simulink library "system_blocks"  (Simulink 8.4)
settings: Solver=ode45  SolverMode=SingleTasking  StartTime=0.0  StopTime=10.0  RelTol=1e-3
values from neighbouring files (symbols this model uses):
  A = 'STP1'    [digital_communications_gui.m]
  D = 'STP4'    [digital_communications_gui.m]
  T = 273+20    (= 293)    [exercise_00.m]
undefined symbols (not defined in the file or in its folder): T4
libraries: simulink x9, dspswit3 x5, dspsigops x2, dspobslib x2, dsparch4 x1, simulink_extras x1, dspmtrx3 x1
(part 1 of 2)
settings Model: Creator=Schoenen  LastModifiedBy=Schoenen

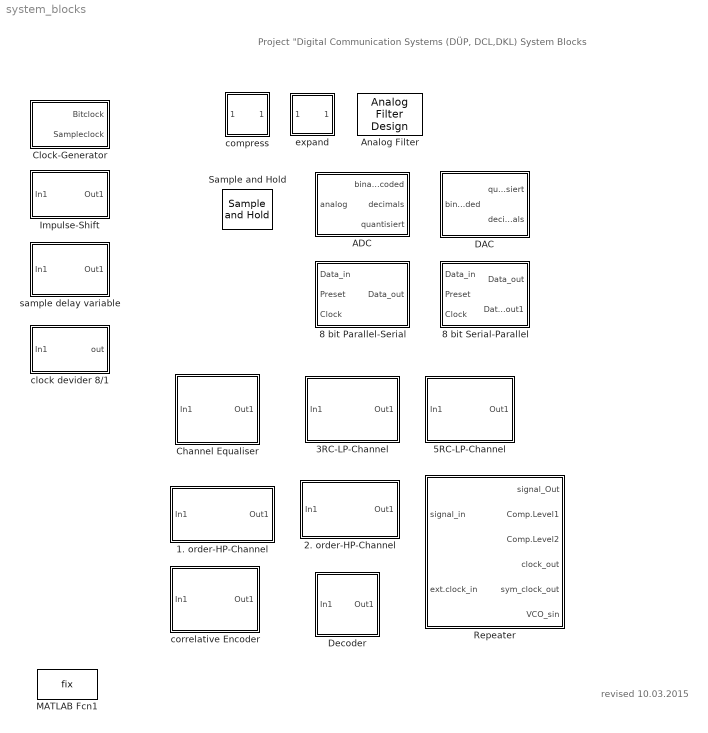
== system system_blocks ==
  note: revised 10.03.2015
  note: Project "Digital Communication Systems (DÜP, DCL,DKL)
      | System Blocks
  1. order-HP-Channel : Subsystem  mask{grenz=400}
      mask prompts: grenz "3 dB-Cutoff frequency (Hz):"
      mask help: Hochpass 1. Ordnung mit wählbarer Grenzfrequenz
      mask init:
      | if grenz==1 T=1/(2*pi*400); end;
      | if grenz==2 T=1/(2*pi*2e3); end;
      | if grenz==3 T=1/(2*pi*3e3); end;
      mask TypeOptions grenz: 400 | 2e3 | 3e3
  2. order-HP-Channel : Subsystem  mask{grenz=400}
      mask prompts: grenz "3 dB-Cutoff frequency (Hz):"
      mask help: Hochpass 2. Ordnung mit wählbarer Grenzfrequenz
      mask init:
      | if grenz==1 T=1/(2*pi*400)*1.554; end;
      | if grenz==2 T=1/(2*pi*2e3)*1.554; end;
      | if grenz==3 T=1/(2*pi*3e3)*1.554; end;
      mask TypeOptions grenz: 400 | 2e3 | 3e3
  "3RC-LP-Channel " : Subsystem  mask{noise=0.1, a=off, step=2/64e5}
      mask prompts: noise "Noise (rms):"; a "Noise on"; step "Simulation Step size:"
      mask help: Kanalmodell mit 3 RC-Gliedern und additivem Rauschen
      mask init:
      | T=10e3*159e-12;
  "5RC-LP-Channel " : Subsystem  mask{noise=0.1, a=off, step=2/64e5}
      mask prompts: noise "Noise (rms):"; a "Noise on"; step "Simulation Step size:"
      mask help: Kanalmodell mit 5 RC-Gliedern und additivem Rauschen
      mask init:
      | T=10e3*159e-12;
  8 bit Parallel-Serial : Subsystem
  8 bit Serial-Parallel : Subsystem
  ADC : Subsystem  mask(Analog-Digital-Converter (ADC)){umax=1, bits=1, bipolar=off}
      mask prompts: umax "Aussteuergrenze:"; bits "Bitanzahl (1...16):"; bipolar "Bipolares binäres Ausgangssignal (binary_coded)"
      mask help:
      | Der ADC wandelt ein bipolares Analogsignal mit den Austeuergrenzen +/- Umax in ein Digitalsignal entsprechender Bitzahl (PCM) um.
      |
      | Oberer Ausgang:      Bit-Parallel-Ausgang, Binäre Zahlenfolge, je Abtastwert ein Zeilenvektor in Binärdarstellung
      |
      | Mittlerer Ausgang:   dem Eingang entsprechender quantisierter positiver Dezimalwert im Bereich 0.... 2^bits -1
      |
      | Unterer Ausgang:    Quantisiertes, bipolares Signal, begrenzt auf +/- Umax, je Abtastwert ein als Skalar
      mask Help:
      | Author: Prof. Dr.-Ing. Peter Kröger
      | copyright 2002
      | <p>
      | Der ADC wandelt ein bipolares Analogsignal mit den Austeuergrenzen +/- Umax in ein Digitalsignal entsprechender Bitzahl (PCM-Signal) um.
      | <p>
      | Oberer Ausgang:     Binäre Zahlenfolge, je Abtastwert ein Zeilenvektor in
      |                                 Binärdarstellung
      | <p>
      | Mittlerer Ausgang:   dem Eingang entsprechender quantisierter positiver                                           Dezimalwert im Bereich 0.... 2^bits -1
      | <p>
      | Unterer Ausgang:    Quantisiertes, bipolares Signal, begrenzt auf +/- Umax,
      |                              je Abtastwert ein als Skalar
  Analog Filter : dsparch4/Analog Filter Design  method=Butterworth  filttype=Lowpass  N=1  Wlo=1  Whi=80  Rp=2  Rs=40
  Channel Equaliser : Subsystem
  Clock-Generator : Subsystem  mask{bt=1, sr=1}
      mask prompts: bt "Bitclock (Hz):"; sr "Sampleclock (Hz):"
      mask help: Clock-Generator
  DAC : Subsystem  mask(Digital-Analog-Converter (DAC)){umax=1, bits=1, bipolar=off}
      mask prompts: umax "maximum voltage limit"; bits "number of bits (1...16)"; bipolar "bipolar binary input sequence"
      mask help:
      | Der DAC wandelt ein binäres Digitalsignal (PCM) in ein bipolares, quantisiertes Analogsignal mit den Austeuergrenzen +/- Umax um.
      |
      | Eingang :              Bit-Paralleleingang, Binäre PCM-Zahlenfolge, je Abtastwert ein Zeilenvektor in Binärdarstellung
      |
      | Oberer  Ausgang:   Quantisiertes, bipolares Signal, begrenzt auf +/- Umax,  je Abtastwert ein als Skalar
      |
      | Unterer Ausgang:   dem Eingang entsprechender positiver  Dezimalwert im Bereich 0.... 2^bits -1
      mask Help:
      | Author: Prof. Dr.-Ing. Peter Kröger
      | copyright 2002
      | <p>
      | 
      | Der DAC wandelt ein binäres Digitalsignal (PCM) in ein bipolares, quantisiertes Analogsignal mit den Austeuergrenzen +/- Umax um.
      | <p>
      | Eingang :                Binäre PCM-Zahlenfolge, je Abtastwert ein Zeilenvektor in
      |                                Binärdarstellung
      | <p>
      | Oberer  Ausgang:   Quantisiertes, bipolares Signal, begrenzt auf +/- Umax,
      |                                je Abtastwert ein als Skalar
      | <p>
      | Unterer Ausgang:   dem Eingang entsprechender positiver  Dezimalwert
      |                                im Bereich 0.... 2^bits -1
  Decoder : Subsystem
  Impulse-Shift : Subsystem  mask{tau=1, width=1, step=2/64e5}
      mask prompts: tau "Phase-Shift [s]"; width "output impulse-width [s]"; step "Simulation Stepsize [s]"
      mask help:
      | Impulse Shift.
      |
      | The Block is triggered on positive edge at input and answers with an output impulse later correspopnding to the Parameter "Phase Shift".
      | The width of the output impuls can be varied.
      | If periodic triggering is applied to the block, the Phase Shift must be less than the trigger period.
  MATLAB Fcn1 : MATLABFcn  MATLABFcn=fix  OutputDimensions=1
  Repeater : Subsystem
  Sample and Hold : dspsigops/Sample and Hold  trig=Rising edge  initCond=0  latchinput=off
  clock devider 8/1 : Subsystem  mask{bt=1, sr=1}
      mask prompts: bt "Bitclock [Hz]"; sr "Sampleclock [Hz]"
      mask help: Clock-Generator
  compress : Subsystem  mask{ck=16}
      mask prompts: ck "comp. factor ck"
      mask help:
      | A-law-compression
      | ck=1	->	 A=1
      | ck=2	->	 A=5.36
      | ck=4	->	 A=14.77
      | ck=8	->	 A=36.85
      | ck=16	->	A=87.56  (ISDN)
      | ck=32	->	A=201.84
      mask init:
      | if ck==1, A=1;
      | 	elseif ck==2, A=5.36;
      | 	elseif ck==4, A=14.77;
      | 	elseif ck==8, A=36.85;
      | 	elseif ck==16, A=87.56;
      | 	else A=201.84;
      | 	end;
      | 	
      | x=-1:.01:1;
      | for i=1:201, 
      | 	if abs(x(i))<1/A, y(i)=ck*x(i); 
      | 	else y(i) = sign(x(i))*(1+log(A*abs(x(i))))/(1+log(A)); 
      | 	end; 
      | end;
      mask Display: plot(x,y)
  correlative Encoder : Subsystem
  expand : Subsystem  mask{ck=16}
      mask prompts: ck "comp. factor ck"
      mask help:
      | A-law-expansion
      | ck=1	->	 A=1
      | ck=2	->	 A=5.36
      | ck=4	->	 A=14.77
      | ck=8	->	 A=36.85
      | ck=16	->	A=87.56  (ISDN)
      | ck=32	->	A=201.84
      mask init:
      | if ck==1, A=1;
      | 	elseif ck==2, A=5.36;
      | 	elseif ck==4, A=14.77;
      | 	elseif ck==8, A=36.85;
      | 	elseif ck==16, A=87.56;
      | 	else A=201.84;
      | 	end;
      | 
      | x=-1:.01:1;
      | for i=1:201,
      | 	if abs(x(i))<ck/A, y(i) = x(i)/ck;
      | 	else y(i) = sign(x(i))*(exp((1+log(A))*abs(x(i)) - 1))/A;
      | 	end;
      | end;
      mask Display: plot(x,y)
  sample delay variable : Subsystem

== system system_blocks/1. order-HP-Channel ==
  In1 : Inport
  HP-1.Ordnung : TransferFcn  Numerator=[T 0]  Denominator=[T 1]
  Out1 : Outport
  wires:
  HP-1.Ordnung/1 -> Out1/1
  In1/1 -> HP-1.Ordnung/1

== system system_blocks/2. order-HP-Channel ==
  In1 : Inport
  HP-1.Ordnung : TransferFcn  Numerator=[T^2 0 0]  Denominator=[T^2 2*T 1]
  Out1 : Outport
  wires:
  HP-1.Ordnung/1 -> Out1/1
  In1/1 -> HP-1.Ordnung/1

== system system_blocks/3RC-LP-Channel  ==
  In1 : Inport
  3 RC-Glieder : TransferFcn  Denominator=[T^3 5*T^2 6*T 1]
  Band-Limited White Noise : Subsystem  mask(Continuous White Noise.){Cov=[noise^2*step], Ts=step, seed=[23341]}
      mask prompts: Cov "Noise Power:"; Ts "Sample Time:"
      mask help:
      | White noise for continuous (s-domain) systems.
      | Band-limited using zero-order-hold.
      mask init:
      | r = rand(1,12); r2 = [r(1),r;r,r(12)]; t =[1:13;1:13];
      mask Help: Implemented using white noise into Zero-Order Hold block. The seed and power can be vectors of the same length to produce a vector of white noise sources. For faster simulation, set sample time to the highest value possible but in accordance with the fastest dynamics of system.
      mask Display: plot(t(:),r2(:))
  Constant : Constant  Value=a
  Ground : Ground
  Sum2 : Sum  SaturateOnIntegerOverflow=on  InputSameDT=on  OutDataTypeStr=Inherit: Same as first input
  Switch : Switch  Threshold=0.5  SaturateOnIntegerOverflow=on
  Out1 : Outport
  wires:
  Ground/1 -> Switch/3
  Constant/1 -> Switch/2
  3 RC-Glieder/1 -> Sum2/1
  Band-Limited White Noise/1(Out_1) -> Switch/1
  In1/1 -> 3 RC-Glieder/1
  Switch/1 -> Sum2/2
  Sum2/1 -> Out1/1

== system system_blocks/5RC-LP-Channel  ==
  In1 : Inport
  5 RC-Glieder : TransferFcn  Denominator=[T^5 9*T^4 28*T^3 35*T^2 15*T 1]
  Band-Limited White Noise : Subsystem  mask(Continuous White Noise.){Cov=[noise^2*step], Ts=step, seed=[23341]}
      mask prompts: Cov "Noise Power:"; Ts "Sample Time:"
      mask help:
      | White noise for continuous (s-domain) systems.
      | Band-limited using zero-order-hold.
      mask init:
      | r = rand(1,12); r2 = [r(1),r;r,r(12)]; t =[1:13;1:13];
      mask Help: Implemented using white noise into Zero-Order Hold block. The seed and power can be vectors of the same length to produce a vector of white noise sources. For faster simulation, set sample time to the highest value possible but in accordance with the fastest dynamics of system.
      mask Display: plot(t(:),r2(:))
  Constant : Constant  Value=a
  Ground : Ground
  Sum2 : Sum  SaturateOnIntegerOverflow=on  InputSameDT=on  OutDataTypeStr=Inherit: Same as first input
  Switch : Switch  Threshold=0.5  SaturateOnIntegerOverflow=on
  Out1 : Outport
  wires:
  Ground/1 -> Switch/3
  Constant/1 -> Switch/2
  5 RC-Glieder/1 -> Sum2/1
  Band-Limited White Noise/1(Out_1) -> Switch/1
  In1/1 -> 5 RC-Glieder/1
  Switch/1 -> Sum2/2
  Sum2/1 -> Out1/1

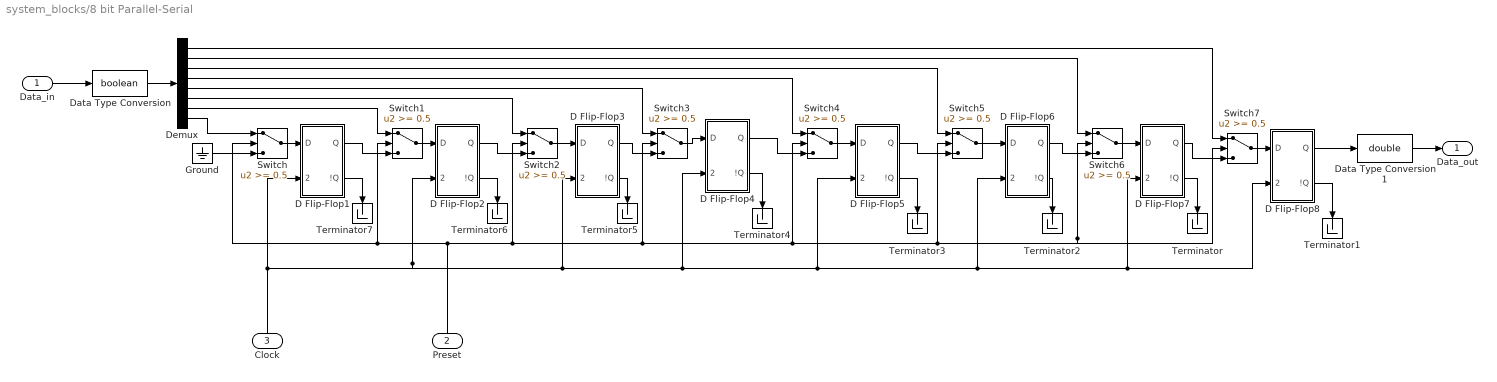
== system system_blocks/8 bit Parallel-Serial ==
  Data_in : Inport
  Preset : Inport  Port=2
  Clock : Inport  Port=3
  D Flip-Flop1 : Subsystem  AncestorBlock=simulink_extras/Flip Flops/D Flip-Flop  mask(DFlipFlop){}
      mask help: D Flip-Flop Block
      mask Help:
      | The D flip-flop block has the following characteristic table:
      | <pre>
      |   Q(t)  D(t)     Q(tnext)
      |   ------------------------
      |    0      0       0
      |    0      1       1
      |    1      0       0
      |    1      1       1
      | </pre>
      | Q(tnext) refers to the output on a clock pulse (CLK) rising edge and when the
      | chip is enabled (!CLR ~= 0).
      | <br><br>
      | The D flip-flop transfers "data" into a memory element (flip-flop) on each clock
      | pulse (CLK). The chip enable input signal, !CLR, is sometimes given the
      | designation G (for gate) to indicate that this input enables the gated latch
      | allowing data entry into the flip-flop.
  D Flip-Flop2 : Subsystem  AncestorBlock=simulink_extras/Flip Flops/D Flip-Flop  mask(DFlipFlop){}
      mask help: D Flip-Flop Block
      mask Help:
      | The D flip-flop block has the following characteristic table:
      | <pre>
      |   Q(t)  D(t)     Q(tnext)
      |   ------------------------
      |    0      0       0
      |    0      1       1
      |    1      0       0
      |    1      1       1
      | </pre>
      | Q(tnext) refers to the output on a clock pulse (CLK) rising edge and when the
      | chip is enabled (!CLR ~= 0).
      | <br><br>
      | The D flip-flop transfers "data" into a memory element (flip-flop) on each clock
      | pulse (CLK). The chip enable input signal, !CLR, is sometimes given the
      | designation G (for gate) to indicate that this input enables the gated latch
      | allowing data entry into the flip-flop.
  D Flip-Flop3 : Subsystem  AncestorBlock=simulink_extras/Flip Flops/D Flip-Flop  mask(DFlipFlop){}
      mask help: D Flip-Flop Block
      mask Help:
      | The D flip-flop block has the following characteristic table:
      | <pre>
      |   Q(t)  D(t)     Q(tnext)
      |   ------------------------
      |    0      0       0
      |    0      1       1
      |    1      0       0
      |    1      1       1
      | </pre>
      | Q(tnext) refers to the output on a clock pulse (CLK) rising edge and when the
      | chip is enabled (!CLR ~= 0).
      | <br><br>
      | The D flip-flop transfers "data" into a memory element (flip-flop) on each clock
      | pulse (CLK). The chip enable input signal, !CLR, is sometimes given the
      | designation G (for gate) to indicate that this input enables the gated latch
      | allowing data entry into the flip-flop.
  D Flip-Flop4 : Subsystem  AncestorBlock=simulink_extras/Flip Flops/D Flip-Flop  mask(DFlipFlop){}
      mask help: D Flip-Flop Block
      mask Help:
      | The D flip-flop block has the following characteristic table:
      | <pre>
      |   Q(t)  D(t)     Q(tnext)
      |   ------------------------
      |    0      0       0
      |    0      1       1
      |    1      0       0
      |    1      1       1
      | </pre>
      | Q(tnext) refers to the output on a clock pulse (CLK) rising edge and when the
      | chip is enabled (!CLR ~= 0).
      | <br><br>
      | The D flip-flop transfers "data" into a memory element (flip-flop) on each clock
      | pulse (CLK). The chip enable input signal, !CLR, is sometimes given the
      | designation G (for gate) to indicate that this input enables the gated latch
      | allowing data entry into the flip-flop.
  D Flip-Flop5 : Subsystem  AncestorBlock=simulink_extras/Flip Flops/D Flip-Flop  mask(DFlipFlop){}
      mask help: D Flip-Flop Block
      mask Help:
      | The D flip-flop block has the following characteristic table:
      | <pre>
      |   Q(t)  D(t)     Q(tnext)
      |   ------------------------
      |    0      0       0
      |    0      1       1
      |    1      0       0
      |    1      1       1
      | </pre>
      | Q(tnext) refers to the output on a clock pulse (CLK) rising edge and when the
      | chip is enabled (!CLR ~= 0).
      | <br><br>
      | The D flip-flop transfers "data" into a memory element (flip-flop) on each clock
      | pulse (CLK). The chip enable input signal, !CLR, is sometimes given the
      | designation G (for gate) to indicate that this input enables the gated latch
      | allowing data entry into the flip-flop.
  D Flip-Flop6 : Subsystem  AncestorBlock=simulink_extras/Flip Flops/D Flip-Flop  mask(DFlipFlop){}
      mask help: D Flip-Flop Block
      mask Help:
      | The D flip-flop block has the following characteristic table:
      | <pre>
      |   Q(t)  D(t)     Q(tnext)
      |   ------------------------
      |    0      0       0
      |    0      1       1
      |    1      0       0
      |    1      1       1
      | </pre>
      | Q(tnext) refers to the output on a clock pulse (CLK) rising edge and when the
      | chip is enabled (!CLR ~= 0).
      | <br><br>
      | The D flip-flop transfers "data" into a memory element (flip-flop) on each clock
      | pulse (CLK). The chip enable input signal, !CLR, is sometimes given the
      | designation G (for gate) to indicate that this input enables the gated latch
      | allowing data entry into the flip-flop.
  D Flip-Flop7 : Subsystem  AncestorBlock=simulink_extras/Flip Flops/D Flip-Flop  mask(DFlipFlop){}
      mask help: D Flip-Flop Block
      mask Help:
      | The D flip-flop block has the following characteristic table:
      | <pre>
      |   Q(t)  D(t)     Q(tnext)
      |   ------------------------
      |    0      0       0
      |    0      1       1
      |    1      0       0
      |    1      1       1
      | </pre>
      | Q(tnext) refers to the output on a clock pulse (CLK) rising edge and when the
      | chip is enabled (!CLR ~= 0).
      | <br><br>
      | The D flip-flop transfers "data" into a memory element (flip-flop) on each clock
      | pulse (CLK). The chip enable input signal, !CLR, is sometimes given the
      | designation G (for gate) to indicate that this input enables the gated latch
      | allowing data entry into the flip-flop.
  D Flip-Flop8 : Subsystem  AncestorBlock=simulink_extras/Flip Flops/D Flip-Flop  mask(DFlipFlop){}
      mask help: D Flip-Flop Block
      mask Help:
      | The D flip-flop block has the following characteristic table:
      | <pre>
      |   Q(t)  D(t)     Q(tnext)
      |   ------------------------
      |    0      0       0
      |    0      1       1
      |    1      0       0
      |    1      1       1
      | </pre>
      | Q(tnext) refers to the output on a clock pulse (CLK) rising edge and when the
      | chip is enabled (!CLR ~= 0).
      | <br><br>
      | The D flip-flop transfers "data" into a memory element (flip-flop) on each clock
      | pulse (CLK). The chip enable input signal, !CLR, is sometimes given the
      | designation G (for gate) to indicate that this input enables the gated latch
      | allowing data entry into the flip-flop.
  Data Type Conversion : DataTypeConversion  OutDataTypeStr=boolean  SaturateOnIntegerOverflow=on  RndMeth=Zero
  Data Type Conversion1 : DataTypeConversion  OutDataTypeStr=double  SaturateOnIntegerOverflow=on  RndMeth=Zero
  Demux : Demux  Outputs=8
  Ground : Ground
  Switch{,1..7} (8 alike) : Switch  Threshold=0.5  SaturateOnIntegerOverflow=on
  Terminator{,1..7} (8 alike) : Terminator
  Data_out : Outport
  wires:
  Data Type Conversion1/1 -> Data_out/1
  D Flip-Flop8/1(Q) -> Data Type Conversion1/1
  Preset/1 -> Switch7/2, Switch6/2, Switch5/2, Switch4/2, Switch3/2, Switch2/2, Switch1/2, Switch/2
  Clock/1 -> D Flip-Flop1/2(CLK), D Flip-Flop2/2(CLK), D Flip-Flop3/2(CLK), D Flip-Flop4/2(CLK), D Flip-Flop5/2(CLK), D Flip-Flop6/2(CLK), D Flip-Flop8/2(CLK), D Flip-Flop7/2(CLK)
  Data_in/1 -> Data Type Conversion/1
  Data Type Conversion/1 -> Demux/1
  D Flip-Flop1/2(!Q) -> Terminator7/1
  D Flip-Flop2/2(!Q) -> Terminator6/1
  D Flip-Flop3/2(!Q) -> Terminator5/1
  D Flip-Flop4/2(!Q) -> Terminator4/1
  D Flip-Flop5/2(!Q) -> Terminator3/1
  D Flip-Flop6/2(!Q) -> Terminator2/1
  D Flip-Flop8/2(!Q) -> Terminator1/1
  D Flip-Flop7/2(!Q) -> Terminator/1
  Demux/1 -> Switch7/1
  Demux/2 -> Switch6/1
  Demux/3 -> Switch5/1
  Demux/4 -> Switch4/1
  Demux/5 -> Switch3/1
  Demux/6 -> Switch2/1
  Demux/7 -> Switch1/1
  Demux/8 -> Switch/1
  D Flip-Flop3/1(Q) -> Switch3/3
  D Flip-Flop7/1(Q) -> Switch7/3
  D Flip-Flop5/1(Q) -> Switch5/3
  Switch7/1 -> D Flip-Flop8/1(D)
  D Flip-Flop6/1(Q) -> Switch6/3
  Switch6/1 -> D Flip-Flop7/1(D)
  Switch5/1 -> D Flip-Flop6/1(D)
  D Flip-Flop4/1(Q) -> Switch4/3
  Switch4/1 -> D Flip-Flop5/1(D)
  Switch3/1 -> D Flip-Flop4/1(D)
  D Flip-Flop2/1(Q) -> Switch2/3
  Switch2/1 -> D Flip-Flop3/1(D)
  Ground/1 -> Switch/3
  D Flip-Flop1/1(Q) -> Switch1/3
  Switch1/1 -> D Flip-Flop2/1(D)
  Switch/1 -> D Flip-Flop1/1(D)

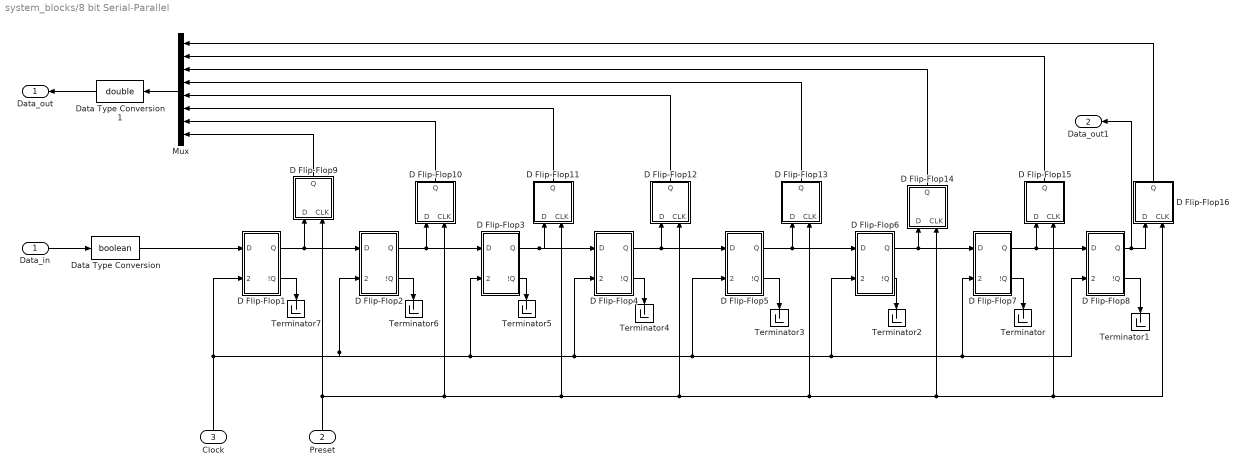
== system system_blocks/8 bit Serial-Parallel ==
  Data_in : Inport
  Preset : Inport  Port=2
  Clock : Inport  Port=3
  D Flip-Flop1 : Subsystem  AncestorBlock=simulink_extras/Flip Flops/D Flip-Flop  mask(DFlipFlop){}
      mask help: D Flip-Flop Block
      mask Help:
      | The D flip-flop block has the following characteristic table:
      | <pre>
      |   Q(t)  D(t)     Q(tnext)
      |   ------------------------
      |    0      0       0
      |    0      1       1
      |    1      0       0
      |    1      1       1
      | </pre>
      | Q(tnext) refers to the output on a clock pulse (CLK) rising edge and when the
      | chip is enabled (!CLR ~= 0).
      | <br><br>
      | The D flip-flop transfers "data" into a memory element (flip-flop) on each clock
      | pulse (CLK). The chip enable input signal, !CLR, is sometimes given the
      | designation G (for gate) to indicate that this input enables the gated latch
      | allowing data entry into the flip-flop.
  D Flip-Flop10 : Subsystem  AncestorBlock=simulink_extras/Flip Flops/D Flip-Flop  mask(DFlipFlop){}
      mask help: D Flip-Flop Block
      mask Help:
      | The D flip-flop block has the following characteristic table:
      | <pre>
      |   Q(t)  D(t)     Q(tnext)
      |   ------------------------
      |    0      0       0
      |    0      1       1
      |    1      0       0
      |    1      1       1
      | </pre>
      | Q(tnext) refers to the output on a clock pulse (CLK) rising edge and when the
      | chip is enabled (!CLR ~= 0).
      | <br><br>
      | The D flip-flop transfers "data" into a memory element (flip-flop) on each clock
      | pulse (CLK). The chip enable input signal, !CLR, is sometimes given the
      | designation G (for gate) to indicate that this input enables the gated latch
      | allowing data entry into the flip-flop.
  D Flip-Flop11 : Subsystem  AncestorBlock=simulink_extras/Flip Flops/D Flip-Flop  mask(DFlipFlop){}
      mask help: D Flip-Flop Block
      mask Help:
      | The D flip-flop block has the following characteristic table:
      | <pre>
      |   Q(t)  D(t)     Q(tnext)
      |   ------------------------
      |    0      0       0
      |    0      1       1
      |    1      0       0
      |    1      1       1
      | </pre>
      | Q(tnext) refers to the output on a clock pulse (CLK) rising edge and when the
      | chip is enabled (!CLR ~= 0).
      | <br><br>
      | The D flip-flop transfers "data" into a memory element (flip-flop) on each clock
      | pulse (CLK). The chip enable input signal, !CLR, is sometimes given the
      | designation G (for gate) to indicate that this input enables the gated latch
      | allowing data entry into the flip-flop.
  D Flip-Flop12 : Subsystem  AncestorBlock=simulink_extras/Flip Flops/D Flip-Flop  mask(DFlipFlop){}
      mask help: D Flip-Flop Block
      mask Help:
      | The D flip-flop block has the following characteristic table:
      | <pre>
      |   Q(t)  D(t)     Q(tnext)
      |   ------------------------
      |    0      0       0
      |    0      1       1
      |    1      0       0
      |    1      1       1
      | </pre>
      | Q(tnext) refers to the output on a clock pulse (CLK) rising edge and when the
      | chip is enabled (!CLR ~= 0).
      | <br><br>
      | The D flip-flop transfers "data" into a memory element (flip-flop) on each clock
      | pulse (CLK). The chip enable input signal, !CLR, is sometimes given the
      | designation G (for gate) to indicate that this input enables the gated latch
      | allowing data entry into the flip-flop.
  D Flip-Flop13 : Subsystem  AncestorBlock=simulink_extras/Flip Flops/D Flip-Flop  mask(DFlipFlop){}
      mask help: D Flip-Flop Block
      mask Help:
      | The D flip-flop block has the following characteristic table:
      | <pre>
      |   Q(t)  D(t)     Q(tnext)
      |   ------------------------
      |    0      0       0
      |    0      1       1
      |    1      0       0
      |    1      1       1
      | </pre>
      | Q(tnext) refers to the output on a clock pulse (CLK) rising edge and when the
      | chip is enabled (!CLR ~= 0).
      | <br><br>
      | The D flip-flop transfers "data" into a memory element (flip-flop) on each clock
      | pulse (CLK). The chip enable input signal, !CLR, is sometimes given the
      | designation G (for gate) to indicate that this input enables the gated latch
      | allowing data entry into the flip-flop.
  D Flip-Flop14 : Subsystem  AncestorBlock=simulink_extras/Flip Flops/D Flip-Flop  mask(DFlipFlop){}
      mask help: D Flip-Flop Block
      mask Help:
      | The D flip-flop block has the following characteristic table:
      | <pre>
      |   Q(t)  D(t)     Q(tnext)
      |   ------------------------
      |    0      0       0
      |    0      1       1
      |    1      0       0
      |    1      1       1
      | </pre>
      | Q(tnext) refers to the output on a clock pulse (CLK) rising edge and when the
      | chip is enabled (!CLR ~= 0).
      | <br><br>
      | The D flip-flop transfers "data" into a memory element (flip-flop) on each clock
      | pulse (CLK). The chip enable input signal, !CLR, is sometimes given the
      | designation G (for gate) to indicate that this input enables the gated latch
      | allowing data entry into the flip-flop.
  D Flip-Flop15 : Subsystem  AncestorBlock=simulink_extras/Flip Flops/D Flip-Flop  mask(DFlipFlop){}
      mask help: D Flip-Flop Block
      mask Help:
      | The D flip-flop block has the following characteristic table:
      | <pre>
      |   Q(t)  D(t)     Q(tnext)
      |   ------------------------
      |    0      0       0
      |    0      1       1
      |    1      0       0
      |    1      1       1
      | </pre>
      | Q(tnext) refers to the output on a clock pulse (CLK) rising edge and when the
      | chip is enabled (!CLR ~= 0).
      | <br><br>
      | The D flip-flop transfers "data" into a memory element (flip-flop) on each clock
      | pulse (CLK). The chip enable input signal, !CLR, is sometimes given the
      | designation G (for gate) to indicate that this input enables the gated latch
      | allowing data entry into the flip-flop.
  D Flip-Flop16 : Subsystem  AncestorBlock=simulink_extras/Flip Flops/D Flip-Flop  mask(DFlipFlop){}
      mask help: D Flip-Flop Block
      mask Help:
      | The D flip-flop block has the following characteristic table:
      | <pre>
      |   Q(t)  D(t)     Q(tnext)
      |   ------------------------
      |    0      0       0
      |    0      1       1
      |    1      0       0
      |    1      1       1
      | </pre>
      | Q(tnext) refers to the output on a clock pulse (CLK) rising edge and when the
      | chip is enabled (!CLR ~= 0).
      | <br><br>
      | The D flip-flop transfers "data" into a memory element (flip-flop) on each clock
      | pulse (CLK). The chip enable input signal, !CLR, is sometimes given the
      | designation G (for gate) to indicate that this input enables the gated latch
      | allowing data entry into the flip-flop.
  D Flip-Flop2 : Subsystem  AncestorBlock=simulink_extras/Flip Flops/D Flip-Flop  mask(DFlipFlop){}
      mask help: D Flip-Flop Block
      mask Help:
      | The D flip-flop block has the following characteristic table:
      | <pre>
      |   Q(t)  D(t)     Q(tnext)
      |   ------------------------
      |    0      0       0
      |    0      1       1
      |    1      0       0
      |    1      1       1
      | </pre>
      | Q(tnext) refers to the output on a clock pulse (CLK) rising edge and when the
      | chip is enabled (!CLR ~= 0).
      | <br><br>
      | The D flip-flop transfers "data" into a memory element (flip-flop) on each clock
      | pulse (CLK). The chip enable input signal, !CLR, is sometimes given the
      | designation G (for gate) to indicate that this input enables the gated latch
      | allowing data entry into the flip-flop.
  D Flip-Flop3 : Subsystem  AncestorBlock=simulink_extras/Flip Flops/D Flip-Flop  mask(DFlipFlop){}
      mask help: D Flip-Flop Block
      mask Help:
      | The D flip-flop block has the following characteristic table:
      | <pre>
      |   Q(t)  D(t)     Q(tnext)
      |   ------------------------
      |    0      0       0
      |    0      1       1
      |    1      0       0
      |    1      1       1
      | </pre>
      | Q(tnext) refers to the output on a clock pulse (CLK) rising edge and when the
      | chip is enabled (!CLR ~= 0).
      | <br><br>
      | The D flip-flop transfers "data" into a memory element (flip-flop) on each clock
      | pulse (CLK). The chip enable input signal, !CLR, is sometimes given the
      | designation G (for gate) to indicate that this input enables the gated latch
      | allowing data entry into the flip-flop.
  D Flip-Flop4 : Subsystem  AncestorBlock=simulink_extras/Flip Flops/D Flip-Flop  mask(DFlipFlop){}
      mask help: D Flip-Flop Block
      mask Help:
      | The D flip-flop block has the following characteristic table:
      | <pre>
      |   Q(t)  D(t)     Q(tnext)
      |   ------------------------
      |    0      0       0
      |    0      1       1
      |    1      0       0
      |    1      1       1
      | </pre>
      | Q(tnext) refers to the output on a clock pulse (CLK) rising edge and when the
      | chip is enabled (!CLR ~= 0).
      | <br><br>
      | The D flip-flop transfers "data" into a memory element (flip-flop) on each clock
      | pulse (CLK). The chip enable input signal, !CLR, is sometimes given the
      | designation G (for gate) to indicate that this input enables the gated latch
      | allowing data entry into the flip-flop.
  D Flip-Flop5 : Subsystem  AncestorBlock=simulink_extras/Flip Flops/D Flip-Flop  mask(DFlipFlop){}
      mask help: D Flip-Flop Block
      mask Help:
      | The D flip-flop block has the following characteristic table:
      | <pre>
      |   Q(t)  D(t)     Q(tnext)
      |   ------------------------
      |    0      0       0
      |    0      1       1
      |    1      0       0
      |    1      1       1
      | </pre>
      | Q(tnext) refers to the output on a clock pulse (CLK) rising edge and when the
      | chip is enabled (!CLR ~= 0).
      | <br><br>
      | The D flip-flop transfers "data" into a memory element (flip-flop) on each clock
      | pulse (CLK). The chip enable input signal, !CLR, is sometimes given the
      | designation G (for gate) to indicate that this input enables the gated latch
      | allowing data entry into the flip-flop.
  D Flip-Flop6 : Subsystem  AncestorBlock=simulink_extras/Flip Flops/D Flip-Flop  mask(DFlipFlop){}
      mask help: D Flip-Flop Block
      mask Help:
      | The D flip-flop block has the following characteristic table:
      | <pre>
      |   Q(t)  D(t)     Q(tnext)
      |   ------------------------
      |    0      0       0
      |    0      1       1
      |    1      0       0
      |    1      1       1
      | </pre>
      | Q(tnext) refers to the output on a clock pulse (CLK) rising edge and when the
      | chip is enabled (!CLR ~= 0).
      | <br><br>
      | The D flip-flop transfers "data" into a memory element (flip-flop) on each clock
      | pulse (CLK). The chip enable input signal, !CLR, is sometimes given the
      | designation G (for gate) to indicate that this input enables the gated latch
      | allowing data entry into the flip-flop.
  D Flip-Flop7 : Subsystem  AncestorBlock=simulink_extras/Flip Flops/D Flip-Flop  mask(DFlipFlop){}
      mask help: D Flip-Flop Block
      mask Help:
      | The D flip-flop block has the following characteristic table:
      | <pre>
      |   Q(t)  D(t)     Q(tnext)
      |   ------------------------
      |    0      0       0
      |    0      1       1
      |    1      0       0
      |    1      1       1
      | </pre>
      | Q(tnext) refers to the output on a clock pulse (CLK) rising edge and when the
      | chip is enabled (!CLR ~= 0).
      | <br><br>
      | The D flip-flop transfers "data" into a memory element (flip-flop) on each clock
      | pulse (CLK). The chip enable input signal, !CLR, is sometimes given the
      | designation G (for gate) to indicate that this input enables the gated latch
      | allowing data entry into the flip-flop.
  D Flip-Flop8 : Subsystem  AncestorBlock=simulink_extras/Flip Flops/D Flip-Flop  mask(DFlipFlop){}
      mask help: D Flip-Flop Block
      mask Help:
      | The D flip-flop block has the following characteristic table:
      | <pre>
      |   Q(t)  D(t)     Q(tnext)
      |   ------------------------
      |    0      0       0
      |    0      1       1
      |    1      0       0
      |    1      1       1
      | </pre>
      | Q(tnext) refers to the output on a clock pulse (CLK) rising edge and when the
      | chip is enabled (!CLR ~= 0).
      | <br><br>
      | The D flip-flop transfers "data" into a memory element (flip-flop) on each clock
      | pulse (CLK). The chip enable input signal, !CLR, is sometimes given the
      | designation G (for gate) to indicate that this input enables the gated latch
      | allowing data entry into the flip-flop.
  D Flip-Flop9 : Subsystem  AncestorBlock=simulink_extras/Flip Flops/D Flip-Flop  mask(DFlipFlop){}
      mask help: D Flip-Flop Block
      mask Help:
      | The D flip-flop block has the following characteristic table:
      | <pre>
      |   Q(t)  D(t)     Q(tnext)
      |   ------------------------
      |    0      0       0
      |    0      1       1
      |    1      0       0
      |    1      1       1
      | </pre>
      | Q(tnext) refers to the output on a clock pulse (CLK) rising edge and when the
      | chip is enabled (!CLR ~= 0).
      | <br><br>
      | The D flip-flop transfers "data" into a memory element (flip-flop) on each clock
      | pulse (CLK). The chip enable input signal, !CLR, is sometimes given the
      | designation G (for gate) to indicate that this input enables the gated latch
      | allowing data entry into the flip-flop.
  Data Type Conversion : DataTypeConversion  OutDataTypeStr=boolean  SaturateOnIntegerOverflow=on  RndMeth=Zero
  Data Type Conversion1 : DataTypeConversion  OutDataTypeStr=double  SaturateOnIntegerOverflow=on  RndMeth=Zero
  Mux : Mux  Inputs=8
  Terminator{,1..7} (8 alike) : Terminator
  Data_out : Outport
  Data_out1 : Outport  Port=2
  wires:
  D Flip-Flop9/1(Q) -> Mux/8
  D Flip-Flop10/1(Q) -> Mux/7
  D Flip-Flop11/1(Q) -> Mux/6
  D Flip-Flop12/1(Q) -> Mux/5
  D Flip-Flop13/1(Q) -> Mux/4
  D Flip-Flop14/1(Q) -> Mux/3
  D Flip-Flop15/1(Q) -> Mux/2
  D Flip-Flop16/1(Q) -> Mux/1
  Data Type Conversion1/1 -> Data_out/1
  Mux/1 -> Data Type Conversion1/1
  D Flip-Flop8/1(Q) -> Data_out1/1, D Flip-Flop16/1(D)
  Preset/1 -> D Flip-Flop16/2(CLK), D Flip-Flop15/2(CLK), D Flip-Flop14/2(CLK), D Flip-Flop13/2(CLK), D Flip-Flop12/2(CLK), D Flip-Flop11/2(CLK), D Flip-Flop10/2(CLK), D Flip-Flop9/2(CLK)
  Data Type Conversion/1 -> D Flip-Flop1/1(D)
  D Flip-Flop7/1(Q) -> D Flip-Flop15/1(D), D Flip-Flop8/1(D)
  D Flip-Flop5/1(Q) -> D Flip-Flop13/1(D), D Flip-Flop6/1(D)
  Clock/1 -> D Flip-Flop1/2(CLK), D Flip-Flop2/2(CLK), D Flip-Flop3/2(CLK), D Flip-Flop4/2(CLK), D Flip-Flop5/2(CLK), D Flip-Flop6/2(CLK), D Flip-Flop8/2(CLK), D Flip-Flop7/2(CLK)
  Data_in/1 -> Data Type Conversion/1
  D Flip-Flop1/2(!Q) -> Terminator7/1
  D Flip-Flop2/2(!Q) -> Terminator6/1
  D Flip-Flop3/2(!Q) -> Terminator5/1
  D Flip-Flop4/2(!Q) -> Terminator4/1
  D Flip-Flop5/2(!Q) -> Terminator3/1
  D Flip-Flop6/2(!Q) -> Terminator2/1
  D Flip-Flop8/2(!Q) -> Terminator1/1
  D Flip-Flop7/2(!Q) -> Terminator/1
  D Flip-Flop3/1(Q) -> D Flip-Flop11/1(D), D Flip-Flop4/1(D)
  D Flip-Flop6/1(Q) -> D Flip-Flop14/1(D), D Flip-Flop7/1(D)
  D Flip-Flop4/1(Q) -> D Flip-Flop12/1(D), D Flip-Flop5/1(D)
  D Flip-Flop2/1(Q) -> D Flip-Flop10/1(D), D Flip-Flop3/1(D)
  D Flip-Flop1/1(Q) -> D Flip-Flop9/1(D), D Flip-Flop2/1(D)

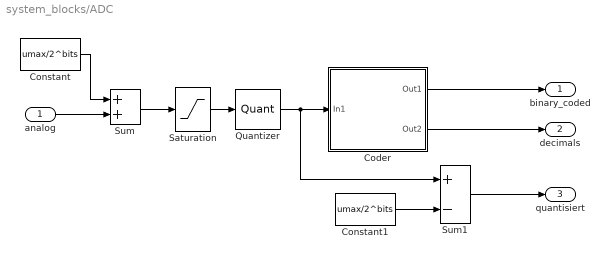
== system system_blocks/ADC ==
  analog : Inport
  Coder : Subsystem
  Constant : Constant  Value=umax/2^bits
  Constant1 : Constant  Value=umax/2^bits
  Quantizer : Quantizer  QuantizationInterval=2*umax/2^bits
  Saturation : Saturate  UpperLimit=umax  LowerLimit=-umax
  Sum : Sum  SaturateOnIntegerOverflow=on  InputSameDT=on  OutDataTypeStr=Inherit: Same as first input
  Sum1 : Sum  Inputs=+-  SaturateOnIntegerOverflow=on  InputSameDT=on  OutDataTypeStr=Inherit: Same as first input
  binary_coded : Outport
  decimals : Outport  Port=2
  quantisiert : Outport  Port=3
  wires:
  Coder/1(Out1) -> binary_coded/1
  Constant1/1 -> Sum1/2
  Quantizer/1 -> Sum1/1, Coder/1(In1)
  Sum1/1 -> quantisiert/1
  Constant/1 -> Sum/1
  Sum/1 -> Saturation/1
  analog/1 -> Sum/2
  Saturation/1 -> Quantizer/1
  Coder/2(Out2) -> decimals/1

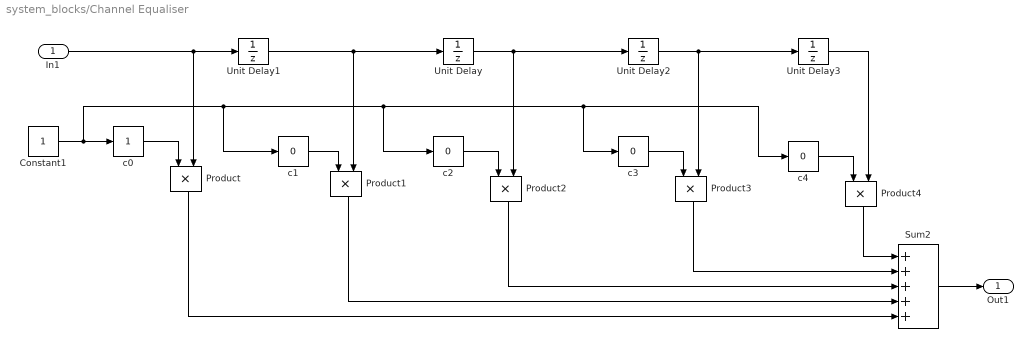
== system system_blocks/Channel Equaliser ==
  In1 : Inport
  Constant1 : Constant
  Product{,1..4} (5 alike) : Product  SaturateOnIntegerOverflow=on  OutDataTypeStr=Inherit: Same as first input
  Sum2 : Sum  Inputs=+++++  SaturateOnIntegerOverflow=on  InputSameDT=on  OutDataTypeStr=Inherit: Same as first input
  Unit Delay{,1..3} (4 alike) : UnitDelay  SampleTime=1/64e3
  c0 : simulink/Math Operations/Slider Gain  low=-1  gain=1  high=1
  c{1..4} (4 alike) : simulink/Math Operations/Slider Gain  low=-1  gain=0  high=1
  Out1 : Outport
  wires:
  Product/1 -> Sum2/5
  Product1/1 -> Sum2/4
  Product2/1 -> Sum2/3
  Product3/1 -> Sum2/2
  Product4/1 -> Sum2/1
  Sum2/1 -> Out1/1
  c4/1 -> Product4/1
  Unit Delay3/1 -> Product4/2
  c3/1 -> Product3/1
  Unit Delay2/1 -> Unit Delay3/1, Product3/2
  c2/1 -> Product2/1
  c1/1 -> Product1/1
  c0/1 -> Product/1
  Constant1/1 -> c4/1, c3/1, c2/1, c1/1, c0/1
  In1/1 -> Product/2, Unit Delay1/1
  Unit Delay/1 -> Unit Delay2/1, Product2/2
  Unit Delay1/1 -> Product1/2, Unit Delay/1

== system system_blocks/Clock-Generator ==
  Clock : simulink_extras/Flip Flops/Clock  period=1/bt
  Constant1 : Constant  Value=bt/sr-1
  Counter : dspswit3/Counter  Direction=Up  CountEvent=Rising edge  CounterSize=User defined  MaxCount=bt/sr-1  InitialCount=0  Output=Count  HitValue=32  ResetInput=off  SamplesPerFrame=1  Ts=1  CntDtype=double  HitDtype=Logical
  Relational Operator : RelationalOperator  Operator===
  Bitclock : Outport
  Sampleclock : Outport  Port=2
  wires:
  Relational Operator/1 -> Sampleclock/1
  Constant1/1 -> Relational Operator/2
  Counter/1 -> Relational Operator/1
  Clock/1 -> Bitclock/1, Counter/1

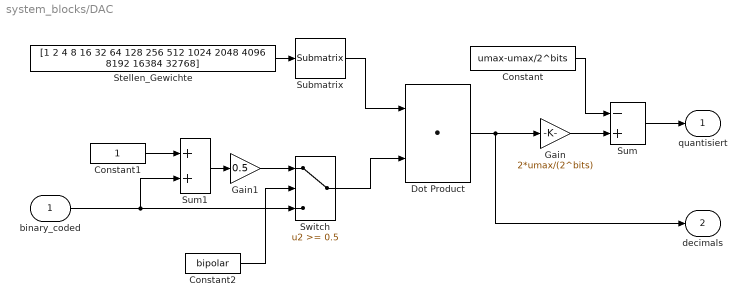
== system system_blocks/DAC ==
  binary_coded : Inport
  Constant : Constant  Value=umax-umax/2^bits
  Constant1 : Constant
  Constant2 : Constant  Value=bipolar
  Dot Product : DotProduct  InputSameDT=on  OutDataTypeStr=Inherit: Inherit via internal rule
  Gain : Gain  Gain=2*umax/(2^bits)  SaturateOnIntegerOverflow=on  OutDataTypeStr=Inherit: Same as input  ParamDataTypeStr=Inherit: Same as input
  Gain1 : Gain  Gain=0.5  SaturateOnIntegerOverflow=on  OutDataTypeStr=Inherit: Same as input  ParamDataTypeStr=Inherit: Same as input
  Stellen_Gewichte : Constant  Value=[1 2 4 8 16 32 64 128 256 512 1024 2048 4096 8192 16384 32768]
  Submatrix : dspmtrx3/Submatrix  RowSpan=Range of rows  RowStartMode=First  RowStartIndex=1  RowEndMode=Index  RowEndIndex=bits  ColSpan=Range of columns  ColStartMode=First  ColStartIndex=1  ColEndMode=Last  ColEndIndex=bits-1
  Sum : Sum  Inputs=-+  SaturateOnIntegerOverflow=on  InputSameDT=on  OutDataTypeStr=Inherit: Same as first input
  Sum1 : Sum  SaturateOnIntegerOverflow=on  InputSameDT=on  OutDataTypeStr=Inherit: Same as first input
  Switch : Switch  Threshold=0.5  SaturateOnIntegerOverflow=on  InputSameDT=on
  quantisiert : Outport
  decimals : Outport  Port=2
  wires:
  Constant2/1 -> Switch/2
  Gain1/1 -> Switch/1
  Sum1/1 -> Gain1/1
  Constant1/1 -> Sum1/1
  binary_coded/1 -> Sum1/2, Switch/3
  Switch/1 -> Dot Product/2
  Gain/1 -> Sum/2
  Dot Product/1 -> decimals/1, Gain/1
  Sum/1 -> quantisiert/1
  Constant/1 -> Sum/1
  Submatrix/1 -> Dot Product/1
  Stellen_Gewichte/1 -> Submatrix/1

== system system_blocks/Decoder ==
  In1 : Inport
  Constant2 : Constant  Value=2
  fcn : Math  Operator=mod  SaturateOnIntegerOverflow=on
  round : MATLABFcn  MATLABFcn=round
  Out1 : Outport
  wires:
  fcn/1 -> Out1/1
  In1/1 -> round/1
  round/1 -> fcn/1
  Constant2/1 -> fcn/2

== system system_blocks/Impulse-Shift ==
  In1 : Inport
  Logical Operator1 : Logic  Operator=NOT  AllPortsSameDT=off
  Monoflop2 : Subsystem  mask{tau=tau, step=step}
      mask prompts: tau "Impulsewidth [s]"; step "Simulation-stepsize"
      mask help:
      | Monoflop
      | positive edge triggered
  Monoflop3 : Subsystem  mask{tau=width, step=step}
      mask prompts: tau "Impulsewidth [s]"; step "Simulation-stepsize"
      mask help:
      | Monoflop
      | positive edge triggered
  Out1 : Outport
  wires:
  Monoflop3/1(Out1) -> Out1/1
  In1/1 -> Monoflop2/1(In1)
  Logical Operator1/1 -> Monoflop3/1(In1)
  Monoflop2/1(Out1) -> Logical Operator1/1

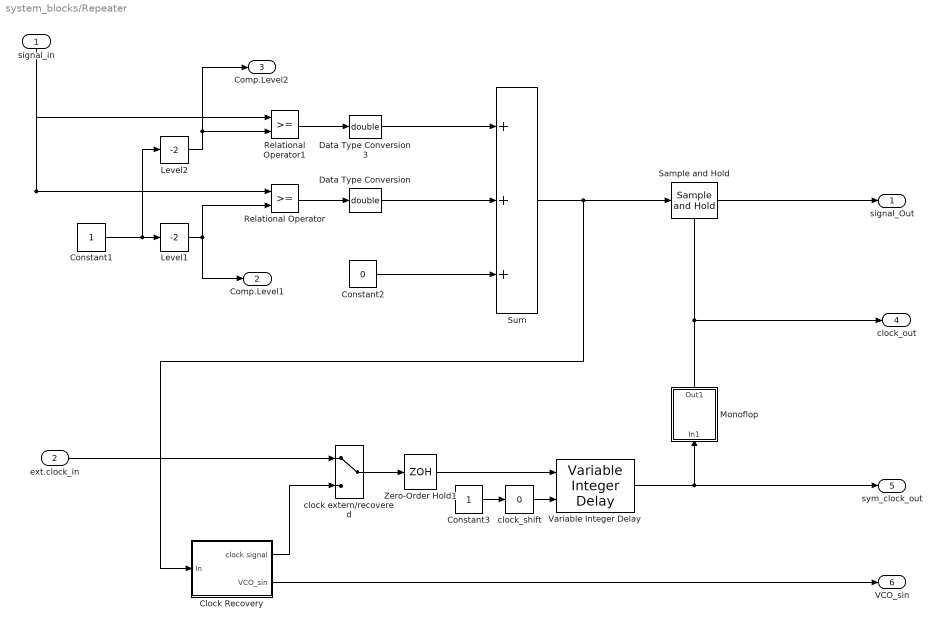
== system system_blocks/Repeater ==
  signal_in : Inport
  ext.clock_in : Inport  Port=2
  Clock Recovery : Subsystem  mask{Typ=Filtergrenzfrequenz : 6Hz, fbit=64e3+0}
      mask prompts: Typ "Schleifenfilter"; fbit "Ruhefrequenz [Hz]"
      mask TypeOptions Typ: Filtergrenzfrequenz : 6Hz | Filtergrenzfrequenz : 20Hz | Filtergrenzfrequenz : 49Hz
  Constant1 : Constant
  Constant2 : Constant  Value=0
  Constant3 : Constant
  Data Type Conversion : DataTypeConversion  OutDataTypeStr=double  SaturateOnIntegerOverflow=on  RndMeth=Zero
  Data Type Conversion3 : DataTypeConversion  OutDataTypeStr=double  SaturateOnIntegerOverflow=on  RndMeth=Zero
  Level1 : simulink/Math Operations/Slider Gain  low=-2  gain=-2  high=2
  Level2 : simulink/Math Operations/Slider Gain  low=-2  gain=-2  high=2
  Monoflop : Subsystem  mask{tau=4/64e5, step=2/64e5}
      mask prompts: tau "Impulsewidth [s]"; step "Simulation-stepsize"
      mask help:
      | Monoflop
      | positive edge triggered
  Relational Operator : RelationalOperator
  Relational Operator1 : RelationalOperator
  Sample and Hold : dspsigops/Sample and Hold  trig=Rising edge  initCond=0  latchinput=off
  Sum : Sum  Inputs=+++  SaturateOnIntegerOverflow=on
  Variable Integer Delay : dspobslib/Variable Integer Delay  dmax=100  InputProcessing=Inherited (this choice will be removed - see release notes)  ic=0  noDFT=off
  Zero-Order Hold1 : ZeroOrderHold  SampleTime=2/64e5
  clock extern/recovered : ManualSwitch
  clock_shift : simulink/Math Operations/Slider Gain  low=0  gain=0  high=100
  signal_Out : Outport
  Comp.Level1 : Outport  Port=2
  Comp.Level2 : Outport  Port=3
  clock_out : Outport  Port=4
  sym_clock_out : Outport  Port=5
  VCO_sin : Outport  Port=6
  wires:
  ext.clock_in/1 -> clock extern/recovered/1
  Clock Recovery/1(clock signal) -> clock extern/recovered/2
  clock extern/recovered/1 -> Zero-Order Hold1/1
  Monoflop/1(Out1) -> clock_out/1, Sample and Hold/Trigger
  Sum/1 -> Sample and Hold/1, Clock Recovery/1(In)
  Data Type Conversion3/1 -> Sum/1
  Data Type Conversion/1 -> Sum/2
  Constant2/1 -> Sum/3
  Zero-Order Hold1/1 -> Variable Integer Delay/1
  Variable Integer Delay/1 -> Monoflop/1(In1), sym_clock_out/1
  Constant3/1 -> clock_shift/1
  clock_shift/1 -> Variable Integer Delay/2
  signal_in/1 -> Relational Operator/1, Relational Operator1/1
  Relational Operator1/1 -> Data Type Conversion3/1
  Relational Operator/1 -> Data Type Conversion/1
  Sample and Hold/1 -> signal_Out/1
  Level2/1 -> Comp.Level2/1, Relational Operator1/2
  Level1/1 -> Comp.Level1/1, Relational Operator/2
  Constant1/1 -> Level2/1, Level1/1
  Clock Recovery/2(VCO_sin) -> VCO_sin/1

== system system_blocks/clock devider 8/1 ==
  In1 : Inport
  Constant1 : Constant  Value=7
  Counter : dspswit3/Counter  Direction=Up  CountEvent=Rising edge  CounterSize=User defined  MaxCount=7  InitialCount=0  Output=Count  HitValue=32  ResetInput=off  SamplesPerFrame=1  Ts=1  CntDtype=double  HitDtype=Logical
  Relational Operator : RelationalOperator  Operator===
  out : Outport
  wires:
  Relational Operator/1 -> out/1
  Constant1/1 -> Relational Operator/2
  Counter/1 -> Relational Operator/1
  In1/1 -> Counter/1

== system system_blocks/compress ==
  In1 : Inport
  S-Function : S-Function  FunctionName=compress  Parameters=ck,A  EnableBusSupport=off
  Out1 : Outport
  wires:
  S-Function/1 -> Out1/1
  In1/1 -> S-Function/1

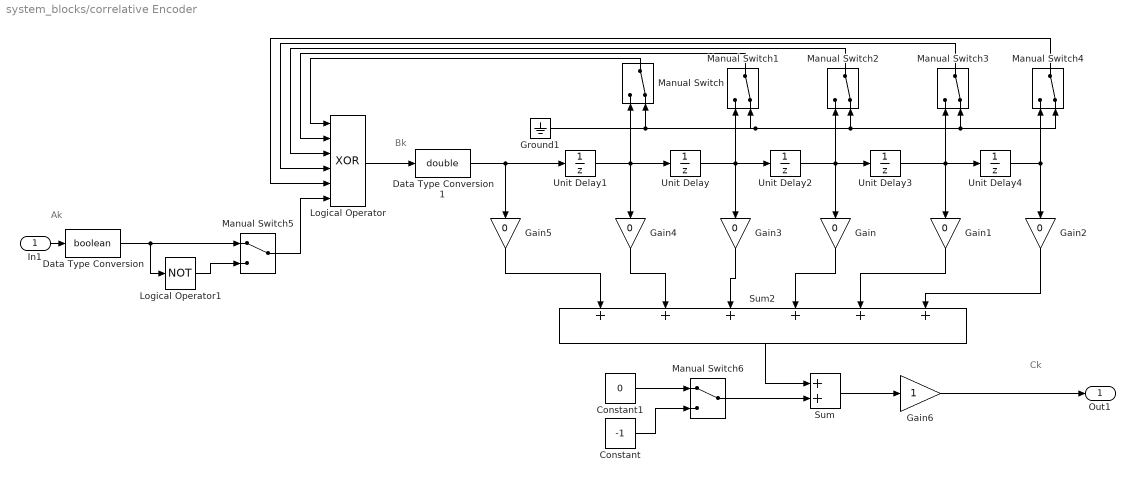
== system system_blocks/correlative Encoder ==
  note: Ak
  note: Bk
  note: Ck
  In1 : Inport
  Constant : Constant  Value=-1
  Constant1 : Constant  Value=0
  Data Type Conversion : DataTypeConversion  OutDataTypeStr=boolean  SaturateOnIntegerOverflow=on  RndMeth=Zero
  Data Type Conversion1 : DataTypeConversion  OutDataTypeStr=double  SaturateOnIntegerOverflow=on  RndMeth=Zero
  Gain{,1..5} (6 alike) : Gain  Gain=0  SaturateOnIntegerOverflow=on  OutDataTypeStr=Inherit: Same as input  ParamDataTypeStr=Inherit: Same as input
  Gain6 : Gain  SaturateOnIntegerOverflow=on  OutDataTypeStr=Inherit: Same as input  ParamDataTypeStr=Inherit: Same as input
  Ground1 : Ground
  Logical Operator : Logic  Operator=XOR  Inputs=6  AllPortsSameDT=off
  Logical Operator1 : Logic  Operator=NOT  AllPortsSameDT=off
  Manual Switch{,1..4} (5 alike) : ManualSwitch  CurrentSetting=0
  Manual Switch5 : ManualSwitch
  Manual Switch6 : ManualSwitch
  Sum : Sum  SaturateOnIntegerOverflow=on
  Sum2 : Sum  Inputs=++++++  SaturateOnIntegerOverflow=on  InputSameDT=on  OutDataTypeStr=Inherit: Same as first input
  Unit Delay{,1..4} (5 alike) : UnitDelay  SampleTime=1/64e3
  Out1 : Outport
  wires:
  Constant/1 -> Manual Switch6/2
  Constant1/1 -> Manual Switch6/1
  Manual Switch6/1 -> Sum/2
  Sum/1 -> Gain6/1
  Sum2/1 -> Sum/1
  Logical Operator1/1 -> Manual Switch5/2
  Manual Switch5/1 -> Logical Operator/6
  Data Type Conversion/1 -> Logical Operator1/1, Manual Switch5/1
  Gain6/1 -> Out1/1
  Ground1/1 -> Manual Switch/2, Manual Switch1/2, Manual Switch2/2, Manual Switch3/2, Manual Switch4/2
  Manual Switch4/1 -> Logical Operator/5
  Manual Switch3/1 -> Logical Operator/4
  Manual Switch2/1 -> Logical Operator/3
  Manual Switch1/1 -> Logical Operator/2
  Manual Switch/1 -> Logical Operator/1
  Data Type Conversion1/1 -> Gain5/1, Unit Delay1/1
  Logical Operator/1 -> Data Type Conversion1/1
  In1/1 -> Data Type Conversion/1
  Gain2/1 -> Sum2/6
  Gain1/1 -> Sum2/5
  Gain/1 -> Sum2/4
  Gain3/1 -> Sum2/3
  Gain4/1 -> Sum2/2
  Gain5/1 -> Sum2/1
  Unit Delay4/1 -> Manual Switch4/1, Gain2/1
  Unit Delay/1 -> Manual Switch1/1, Gain3/1, Unit Delay2/1
  Unit Delay2/1 -> Manual Switch2/1, Gain/1, Unit Delay3/1
  Unit Delay3/1 -> Manual Switch3/1, Gain1/1, Unit Delay4/1
  Unit Delay1/1 -> Manual Switch/1, Gain4/1, Unit Delay/1

== system system_blocks/expand ==
  In1 : Inport
  S-Function : S-Function  FunctionName=expand  Parameters=ck,A  EnableBusSupport=off
  Out1 : Outport
  wires:
  In1/1 -> S-Function/1
  S-Function/1 -> Out1/1

== system system_blocks/sample delay variable ==
  In1 : Inport
  Constant3 : Constant
  Slider Gain : simulink/Math Operations/Slider Gain  low=0  gain=15  high=100
  Variable Integer Delay1 : dspobslib/Variable Integer Delay  dmax=100  InputProcessing=Inherited (this choice will be removed - see release notes)  ic=0  noDFT=off
  Zero-Order Hold1 : ZeroOrderHold  SampleTime=2/64e5
  Out1 : Outport
  wires:
  Variable Integer Delay1/1 -> Out1/1
  In1/1 -> Zero-Order Hold1/1
  Zero-Order Hold1/1 -> Variable Integer Delay1/1
  Constant3/1 -> Slider Gain/1
  Slider Gain/1 -> Variable Integer Delay1/2

== system system_blocks/3RC-LP-Channel /Band-Limited White Noise ==
  Gain : Gain  Gain=[sqrt(Cov)]/[sqrt(Ts)]  SaturateOnIntegerOverflow=on  OutDataTypeStr=Inherit: Same as input  ParamDataTypeStr=Inherit: Same as input
  White Noise : RandomNumber  Seed=seed  SampleTime=Ts
  Zero-Order Hold : ZeroOrderHold  SampleTime=Ts
  Out_1 : Outport
  wires:
  White Noise/1 -> Zero-Order Hold/1
  Gain/1 -> Out_1/1
  Zero-Order Hold/1 -> Gain/1

== system system_blocks/5RC-LP-Channel /Band-Limited White Noise ==
  Gain : Gain  Gain=[sqrt(Cov)]/[sqrt(Ts)]  SaturateOnIntegerOverflow=on  OutDataTypeStr=Inherit: Same as input  ParamDataTypeStr=Inherit: Same as input
  White Noise : RandomNumber  Seed=seed  SampleTime=Ts
  Zero-Order Hold : ZeroOrderHold  SampleTime=Ts
  Out_1 : Outport
  wires:
  White Noise/1 -> Zero-Order Hold/1
  Gain/1 -> Out_1/1
  Zero-Order Hold/1 -> Gain/1

== system system_blocks/8 bit Parallel-Serial/D Flip-Flop1 ==
  D : Inport
  CLK : Inport  Port=2
  Constant1 : Constant
  D Flip-Flop : Subsystem  TreatAsAtomicUnit=on
  Data Type Conversion : DataTypeConversion  OutDataTypeStr=boolean  SaturateOnIntegerOverflow=on  RndMeth=Zero
  Q : Outport  InitialOutput=0
  !Q : Outport  Port=2  InitialOutput=1
  wires:
  Constant1/1 -> Data Type Conversion/1
  Data Type Conversion/1 -> D Flip-Flop/Enable
  CLK/1 -> D Flip-Flop/Trigger
  D Flip-Flop/1(Q) -> Q/1
  D/1 -> D Flip-Flop/1(D)
  D Flip-Flop/2(!Q) -> !Q/1

== system system_blocks/8 bit Parallel-Serial/D Flip-Flop2 ==
  D : Inport
  CLK : Inport  Port=2
  Constant1 : Constant
  D Flip-Flop : Subsystem  TreatAsAtomicUnit=on
  Data Type Conversion : DataTypeConversion  OutDataTypeStr=boolean  SaturateOnIntegerOverflow=on  RndMeth=Zero
  Q : Outport  InitialOutput=0
  !Q : Outport  Port=2  InitialOutput=1
  wires:
  Constant1/1 -> Data Type Conversion/1
  Data Type Conversion/1 -> D Flip-Flop/Enable
  CLK/1 -> D Flip-Flop/Trigger
  D Flip-Flop/1(Q) -> Q/1
  D/1 -> D Flip-Flop/1(D)
  D Flip-Flop/2(!Q) -> !Q/1

== system system_blocks/8 bit Parallel-Serial/D Flip-Flop3 ==
  D : Inport
  CLK : Inport  Port=2
  Constant1 : Constant
  D Flip-Flop : Subsystem  TreatAsAtomicUnit=on
  Data Type Conversion : DataTypeConversion  OutDataTypeStr=boolean  SaturateOnIntegerOverflow=on  RndMeth=Zero
  Q : Outport  InitialOutput=0
  !Q : Outport  Port=2  InitialOutput=1
  wires:
  Constant1/1 -> Data Type Conversion/1
  Data Type Conversion/1 -> D Flip-Flop/Enable
  CLK/1 -> D Flip-Flop/Trigger
  D Flip-Flop/1(Q) -> Q/1
  D/1 -> D Flip-Flop/1(D)
  D Flip-Flop/2(!Q) -> !Q/1

== system system_blocks/8 bit Parallel-Serial/D Flip-Flop4 ==
  D : Inport
  CLK : Inport  Port=2
  Constant1 : Constant
  D Flip-Flop : Subsystem  TreatAsAtomicUnit=on
  Data Type Conversion : DataTypeConversion  OutDataTypeStr=boolean  SaturateOnIntegerOverflow=on  RndMeth=Zero
  Q : Outport  InitialOutput=0
  !Q : Outport  Port=2  InitialOutput=1
  wires:
  Constant1/1 -> Data Type Conversion/1
  Data Type Conversion/1 -> D Flip-Flop/Enable
  CLK/1 -> D Flip-Flop/Trigger
  D Flip-Flop/1(Q) -> Q/1
  D/1 -> D Flip-Flop/1(D)
  D Flip-Flop/2(!Q) -> !Q/1
